simulink model "step5_forward_dyn_kine"  (Simulink 10.2)
settings: Solver=FixedStepAuto  StartTime=0.0  StopTime=3  FixedStep=T_step  RelTol=1e-3
values from neighbouring files (symbols this model uses):
  Coefddq1 = polyfit(tv,ddq1d,5)    [TrajectoryPlanning_simulink.m]    (also in step2.mat = [4.72491967588e-15 -3.27046494167e-13 33.9277839628 -50.8916; step2_trajectory.m = polyfit(t_action,ddq1d,5); step3.m)
  Coefddq2 = polyfit(tv,ddq2d,5)    [TrajectoryPlanning_simulink.m]    (also in step2.mat = [9.35976668804e-13 -4.53899397056e-12 272.296235919 -408.444; step2_trajectory.m = polyfit(t_action,ddq2d,5); step3.m)
  Coefddq3 = polyfit(tv,ddq3d,5)    [TrajectoryPlanning_simulink.m]    (also in step2.mat = [-8.62483792285e-13 3.31083832504e-12 -180.560313738 270.840; step2_trajectory.m = polyfit(t_action,ddq3d,5); step3.m)
  Coefdq1 = polyfit(tv,dq1d,5)    [TrajectoryPlanning_simulink.m]    (also in step2.mat = [-5.68315943596e-14 8.48194599071 -16.9638919814 8.481945990; step2_trajectory.m = polyfit(t_action,dq1d,5); step3.m)
  Coefdq2 = polyfit(tv,dq2d,5)    [TrajectoryPlanning_simulink.m]    (also in step2.mat = [-5.14425222069e-13 68.0740589798 -136.14811796 68.074058979; step2_trajectory.m = polyfit(t_action,dq2d,5); step3.m)
  Coefdq3 = polyfit(tv,dq3d,5)    [TrajectoryPlanning_simulink.m]    (also in step2.mat = [8.05653713588e-13 -45.1400784346 90.2801568692 -45.14007843; step2_trajectory.m = polyfit(t_action,dq3d,5); step3.m)
  Coefq1 = polyfit(tv,q1d,5)    [TrajectoryPlanning_simulink.m]    (also in step2.mat = [1.69638919814 -4.24097299536 2.82731533024 7.50224544818e-1; step2_trajectory.m = polyfit(t_action,q1d,5); step3.m)
  Coefq2 = polyfit(tv,q2d,5)    [TrajectoryPlanning_simulink.m]    (also in step2.mat = [13.614811796 -34.0370294899 22.6913529933 -2.13681015439e-1; step2_trajectory.m = polyfit(t_action,q2d,5); step3.m)
  Coefq3 = polyfit(tv,q3d,5)    [TrajectoryPlanning_simulink.m]    (also in step2.mat = [-9.02801568692 22.5700392173 -15.0466928115 8.32884443522e-; step2_trajectory.m = polyfit(t_action,q3d,5); step3.m)
  F = [Fx;Fy;Mz]    [Jacobi_T.m]    (also in PRBDM_CTC_task.m = M_tilda*v+C_tilda*dX+G_tilda; RRR_CTC_task.m = M_tilda*v+V_tilda*dX+G_tilda; RRR_jtraj.m = q0; step2.mat = 10)
  gama0 = Rparams4dyn(3)    [PRBDM_3R_Dynamic_Matrices_Lagrange.m]    (also in PRBDM_3R_Dynamics.m = in4dyn(12); PRBDM_3R_Dynamics00.m = in4dyn(12); PRBDM_3R_DynamicsPID.m = in4dyn(12); PRBDM_3R_parameters.m = 0.1)
  gama1 = x(7)    [Jacobi_T.m]    (also in PRBDM_3R_Dynamic_Matrices_Lagrange.m = Rparams4dyn(4); PRBDM_3R_Dynamics.m = in4dyn(13); PRBDM_3R_Dynamics00.m = in4dyn(13); PRBDM_3R_DynamicsPID.m = in4dyn(13))
  gama2 = x(8)    [Jacobi_T.m]    (also in PRBDM_3R_Dynamic_Matrices_Lagrange.m = Rparams4dyn(5); PRBDM_3R_Dynamics.m = in4dyn(14); PRBDM_3R_Dynamics00.m = in4dyn(14); PRBDM_3R_DynamicsPID.m = in4dyn(14))
  gama3 = x(9)    [Jacobi_T.m]    (also in PRBDM_3R_Dynamic_Matrices_Lagrange.m = Rparams4dyn(6); PRBDM_3R_Dynamics.m = in4dyn(15); PRBDM_3R_Dynamics00.m = in4dyn(15); PRBDM_3R_DynamicsPID.m = in4dyn(15))
  I = Rparams4dyn(10)    [PRBDM_3R_Dynamic_Matrices_Lagrange.m]    (also in PRBDM_3R_Dynamics.m = in4dyn(19); PRBDM_3R_Dynamics00.m = in4dyn(19); PRBDM_3R_DynamicsPID.m = in4dyn(19); PRBDM_3R_parameters.m = 1.8e-11)
  k1 = Rparams4dyn(7)    [PRBDM_3R_Dynamic_Matrices_Lagrange.m]    (also in PRBDM_3R_Dynamics.m = in4dyn(16); PRBDM_3R_Dynamics00.m = in4dyn(16); PRBDM_3R_DynamicsPID.m = in4dyn(16); PRBDM_3R_parameters.m = 0.290628)
  k2 = Rparams4dyn(8)    [PRBDM_3R_Dynamic_Matrices_Lagrange.m]    (also in PRBDM_3R_Dynamics.m = in4dyn(17); PRBDM_3R_Dynamics00.m = in4dyn(17); PRBDM_3R_DynamicsPID.m = in4dyn(17); PRBDM_3R_parameters.m = 0.247572)
  k3 = Rparams4dyn(9)    [PRBDM_3R_Dynamic_Matrices_Lagrange.m]    (also in PRBDM_3R_Dynamics.m = in4dyn(18); PRBDM_3R_Dynamics00.m = in4dyn(18); PRBDM_3R_DynamicsPID.m = in4dyn(18); PRBDM_3R_parameters.m = 0.213624)
  L = Rparams4dyn(2)    [PRBDM_3R_Dynamic_Matrices_Lagrange.m]    (also in PRBDM_3R_Dynamics.m = in4dyn(11); PRBDM_3R_Dynamics00.m = in4dyn(11); PRBDM_3R_DynamicsPID.m = in4dyn(11); PRBDM_3R_parameters.m = 0.3)
  L0 = z(7)    [Forward_kinematics.m]    (also in GeometricCalculation_simulink.m = Geoparams(4); PRBDM_3R_parameters.m = 0.03; PRBDM_3R_parameters.mat = 0.03; TrajectoryPlanning_simulink.m = X(8))
  L1 = z(8)    [Forward_kinematics.m]    (also in GeometricCalculation_simulink.m = Geoparams(5); Jacobi.m = x(4); PRBDM_3R_CTC.m = x(19); PRBDM_3R_Dynamic_Matrices_NewtonEular.m = robot_params(4))
  L2 = z(9)    [Forward_kinematics.m]    (also in GeometricCalculation_simulink.m = Geoparams(6); Jacobi.m = x(5); PRBDM_3R_CTC.m = x(20); PRBDM_3R_Dynamic_Matrices_NewtonEular.m = robot_params(5))
  L3 = z(10)    [Forward_kinematics.m]    (also in GeometricCalculation_simulink.m = Geoparams(7); Jacobi.m = x(6); PRBDM_3R_CTC.m = x(21); PRBDM_3R_Dynamic_Matrices_NewtonEular.m = robot_params(6))
  m = Rparams4dyn(1)    [PRBDM_3R_Dynamic_Matrices_Lagrange.m]    (also in PRBDM_3R_Dynamics.m = in4dyn(10); PRBDM_3R_Dynamics00.m = in4dyn(10); PRBDM_3R_DynamicsPID.m = in4dyn(10); PRBDM_3R_parameters.m = 1)
  Mz = x(6)    [Jacobi_T.m]    (also in step2.mat = 10; step2_trajectory.m = 10; step3.m = 10)
  phi_f = 1.0471975512    [step2.mat]    (also in step2_trajectory.m; step3.m)
  T_action = 1    [step2.mat]    (also in step2_trajectory.m)
  Theta_init = [0 0 0 0]    [step2.mat]    (also in step2_trajectory.m = [0     0     0     0    ]; step3.m = [0     0     0     0    ])
  W = x(22)    [PRBDM_3R_CTC.m]    (also in PRBDM_3R_Dynamic_Matrices_NewtonEular.m = robot_params(7); PRBDM_3R_Dynamics.m = in4dyn(20); PRBDM_3R_Dynamics00.m = in4dyn(20); PRBDM_3R_DynamicsPID.m = in4dyn(20))
  x_f = 0.0536    [step2.mat]    (also in step2_trajectory.m; step3.m)
  y_f = 0.135    [step2.mat]    (also in step2_trajectory.m; step3.m)
settings Model: Creator=Master  LastModifiedBy=Master
settings SolverCC: AlgebraicLoopSolver=LineSearch
settings DataIOCC: SaveFormat=Dataset  SignalLoggingSaveFormat=Dataset  ReturnWorkspaceOutputs=on
settings OptimizationCC: LifeSpan=auto
settings DebuggingCC: UnderspecifiedInitializationDetection=Simplified  MergeDetectMultiDrivingBlocksExec=error  FcnCallInpInsideContextMsg=error  SFUnexpectedBacktrackingDiag=error  SFNoUnconditionalDefaultTransitionDiag=error  SFExecutionAtInitializationDiag=warning  UnderSpecifiedDimensionMsg=error  ArithmeticOperatorsInVariantConditions=error
settings HardwareCC: ProdBitPerPointer=64  ProdBitPerSizeT=64  ProdBitPerPtrDiffT=64  ProdLargestAtomicFloat=Float  ProdIntDivRoundTo=Zero  ProdEndianess=LittleEndian  ProdWordSize=64  ProdHWDeviceType=Intel->x86-64 (Windows64)
settings ModelReferenceCC: PropagateSignalLabelsOutOfModel=on
settings SFSimCC: SimUseLocalCustomCode=on  CustomCodeUndefinedFunction=FilterOut
settings RTWCC: RTWUseLocalCustomCode=on
settings CodeAppCC: StateflowObjectComments=off
settings GRTTargetCC: TargetLangStandard=C99 (ISO)  CombineOutputUpdateFcns=on  GRTInterface=off
settings ConfigComp: CovMetricSettings=dwe  CovSaveCumulativeToWorkspaceVar=off  CovSaveSingleToWorkspaceVar=off  CovExternalEMLEnable=on

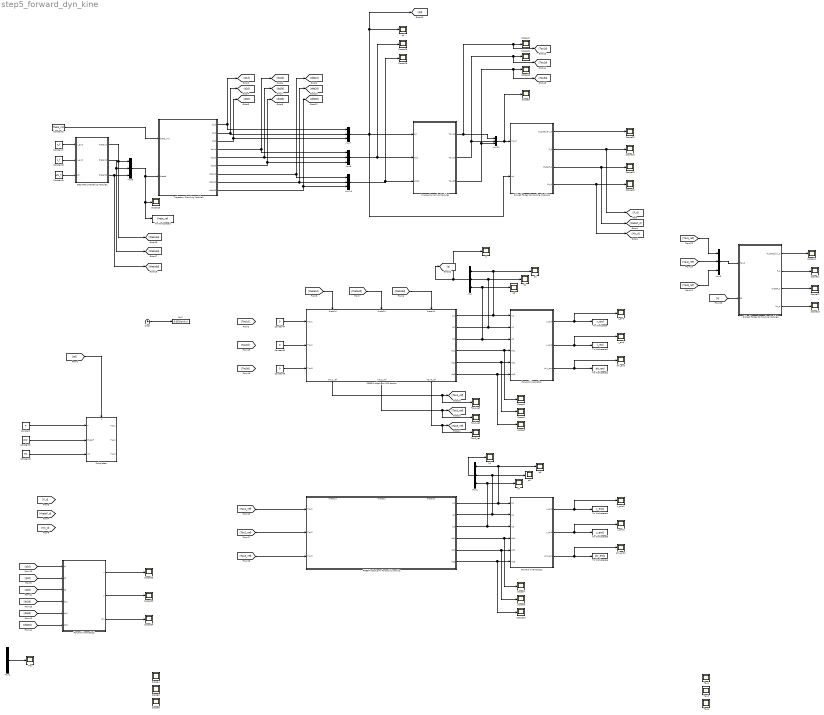
== system step5_forward_dyn_kine ==
  Clock : Clock
  Constant : Constant  Value=F
  Constant1 : Constant  Value=pi/2
  Constant2 : Constant  Value=Theta_init
  Constant3 : Constant  Value=Mz
  Constant4 : Constant  Value=0
  Constant5 : Constant  Value=0
  Constant6 : Constant  Value=0
  Constant7 : Constant  Value=x_f
  Constant8 : Constant  Value=y_f
  Constant9 : Constant  Value=phi_f
  Disired Forces Computing Module1 : Subsystem
  Disired Forces Computing Module2 : Subsystem
  Fcn7 : Fcn  Expr=0.001*sin(u)
  Forward kinematics : Subsystem
  Forward kinematics1 : Subsystem
  Forward kinematics2 : Subsystem
  Geometric Modeling Module1 : Subsystem
  Inverse Dynamics Module1 : Subsystem
  Mux{,1,3,7..11} (8 alike) : Mux  Inputs=3
  Mux2 : Mux  Inputs=6
  PRBDM robot arm Forward dynamics : Subsystem
      settings: PortSchema="{\"entries\":[{\"content\":{\"sides\":[{\"content\":{\"connectorIds\":[\"In1\",\"In2\",\"In3\"]},\"type\":\"ConnectorPlacement.EquallySpacedRectSide\",\"uuid\":\"1f88892b-0bd0-49de-aca9-2c32e7693572\"},{\"content\":{\"connectorIds\":[\"Out1\",\"Out2\",\"Out3\",\"Out4\",\"Out5\",\"Out6\"],\"side\":\"RIGHT\"},\"type\":\"ConnectorPlacement.EquallySpacedRectSide\",\"uuid\":\"b703a21d-fa56-4217-8064-1c2098ab3c38\"},{\"content\":{\"connectorIds\":[\"In4\",\"In5\",\"In6\"],\"side\":\"TOP\"},\"type\":\"ConnectorPlacement.EquallySpacedRectSide\",\"uuid\":\"2526ef97-18a1-4ac3-963d-0ba7d1a2d319\"},{\"content\":{\"connectorIds\":[],\"side\":\"BOTTOM\"},\"type\":\"ConnectorPlacement.EquallySpacedRectSide\",\"uuid\":\"f33fbcfd-8e0b-408f-a669-776188a4cff3\"},{\"content\":{\"connectorIds\":[],\"side\":\"HIDDEN\"},\"type\":\"ConnectorPlacement.EquallySpacedRectSide\",\"uuid\":\"8c9044ff-40c0-4995-b32e-bf50be4b71db\"}]},\"type\":\"ConnectorPlacement.EquallySpacedConnector\",\"uuid\":\"32b5ad01-d59a-45fa-aad8-e0a4c9d304fb\"}],\"packageUris\":[\"http://schema.mathworks.com/mf0/Connector/R2020b\"],\"version\":\"1.0\"}"
      mask Display: image(imread('RRR.png'))
  PRBDM robot arm PID control : Subsystem
      settings: PortSchema="{\"entries\":[{\"content\":{\"sides\":[{\"content\":{\"connectorIds\":[\"In1\",\"In2\",\"In3\"]},\"type\":\"ConnectorPlacement.EquallySpacedRectSide\",\"uuid\":\"1f88892b-0bd0-49de-aca9-2c32e7693572\"},{\"content\":{\"connectorIds\":[\"Out1\",\"Out2\",\"Out3\",\"Out4\",\"Out5\",\"Out6\"],\"side\":\"RIGHT\"},\"type\":\"ConnectorPlacement.EquallySpacedRectSide\",\"uuid\":\"b703a21d-fa56-4217-8064-1c2098ab3c38\"},{\"content\":{\"connectorIds\":[\"In4\",\"In5\",\"In6\"],\"side\":\"TOP\"},\"type\":\"ConnectorPlacement.EquallySpacedRectSide\",\"uuid\":\"2526ef97-18a1-4ac3-963d-0ba7d1a2d319\"},{\"content\":{\"connectorIds\":[\"Out7\",\"Out8\",\"Out9\"],\"side\":\"BOTTOM\"},\"type\":\"ConnectorPlacement.EquallySpacedRectSide\",\"uuid\":\"f33fbcfd-8e0b-408f-a669-776188a4cff3\"},{\"content\":{\"connectorIds\":[],\"side\":\"HIDDEN\"},\"type\":\"ConnectorPlacement.EquallySpacedRectSide\",\"uuid\":\"8c9044ff-40c0-4995-b32e-bf50be4b71db\"}]},\"type\":\"ConnectorPlacement.EquallySpacedConnector\",\"uuid\":\"32b5ad01-d59a-45fa-aad8-e0a4c9d304fb\"}],\"packageUris\":[\"http://schema.mathworks.com/mf0/Connector/R2020b\"],\"version\":\"1.0\"}"
      mask Display: image(imread('RRR.png'))
  Scope{1..14,16..23,25..26,33..35} (27 alike) : Scope
  Subsystem : Subsystem
      settings: PortSchema="{\"entries\":[{\"content\":{\"sides\":[{\"content\":{\"connectorIds\":[\"In1\",\"In2\",\"In3\"]},\"type\":\"ConnectorPlacement.EquallySpacedRectSide\",\"uuid\":\"03e3fa68-98df-40a7-88fb-f274e89646de\"},{\"content\":{\"connectorIds\":[\"Out1\",\"Out2\",\"Out3\"],\"side\":\"RIGHT\"},\"type\":\"ConnectorPlacement.EquallySpacedRectSide\",\"uuid\":\"1a7c6e69-d785-4f03-b0d8-74a38f8f42a1\"},{\"content\":{\"connectorIds\":[\"In4\"],\"side\":\"TOP\"},\"type\":\"ConnectorPlacement.EquallySpacedRectSide\",\"uuid\":\"61c135cb-8cc5-493d-9c37-8230cda997e1\"},{\"content\":{\"connectorIds\":[],\"side\":\"HIDDEN\"},\"type\":\"ConnectorPlacement.EquallySpacedRectSide\",\"uuid\":\"5d99950e-feb6-474c-993a-cad470b06503\"}]},\"type\":\"ConnectorPlacement.EquallySpacedConnector\",\"uuid\":\"5533c5e9-db4a-4e3a-8115-8d67f8979e0c\"}],\"packageUris\":[\"http://schema.mathworks.com/mf0/Connector/R2020b\"],\"version\":\"1.0\"}"
  Tau{,4..6} (4 alike) : Scope
  Tau1_ref : Scope
  Tau2_ref : Scope
  Tau3_ref : Scope
  To Workspace : ToWorkspace  VariableName=x_end  SampleTime=-1
  To Workspace1 : ToWorkspace  VariableName=y_end  SampleTime=-1
  To Workspace2 : ToWorkspace  VariableName=phi_end  SampleTime=-1
  To Workspace3 : ToWorkspace  VariableName=theta_ref  SaveFormat=Timeseries  SampleTime=-1
  To Workspace4 : ToWorkspace  VariableName=x_end1  SampleTime=-1
  To Workspace5 : ToWorkspace  VariableName=y_end1  SampleTime=-1
  To Workspace6 : ToWorkspace  VariableName=phi_end1  SampleTime=-1
  Trajectory Planning Module1 : Subsystem
  phi_end : Scope
  phi_end1 : Scope
  q{,1..7} (8 alike) : Scope
  qd : Scope
  x_end : Scope
  x_end1 : Scope
  y_end : Scope
  y_end1 : Scope
  wires:
  Disired Forces Computing Module1/1(F_cartesian_d) -> Scope23/1
  Constant8/1 -> Geometric Modeling Module1/2(y_end)
  Trajectory Planning Module1/6(dq3d) -> [dq3d], Mux8/3
  Trajectory Planning Module1/9(ddq3d) -> [ddq3d], Mux10/3
  Trajectory Planning Module1/8(ddq2d) -> Mux10/2, [ddq2d]
  Constant9/1 -> Geometric Modeling Module1/3(phi)
  Trajectory Planning Module1/2(q2d) -> Mux7/2, [q2d]
  Trajectory Planning Module1/3(q3d) -> Mux7/3, [q3d]
  Mux11/1 -> Scope8/1, Disired Forces Computing Module1/1(Taud)
  Geometric Modeling Module1/2(theta2d) -> [theta2d], Mux9/2
  Geometric Modeling Module1/1(theta1d) -> [theta1d], Mux9/1
  Mux10/1 -> Inverse Dynamics Module1/3(ddqd), Scope26/1
  Geometric Modeling Module1/3(theta3d) -> [theta3d], Mux9/3
  Mux8/1 -> Inverse Dynamics Module1/2(dqd), Scope25/1
  Trajectory Planning Module1/1(q1d) -> Mux7/1, [q1d]
  Mux9/1 -> To Workspace3/1, Scope16/1, Trajectory Planning Module1/2(thetad)
  Constant7/1 -> Geometric Modeling Module1/1(x_end)
  Constant2/1 -> Trajectory Planning Module1/1(theta_init)
  Inverse Dynamics Module1/1(Tau1d) -> Mux11/1, [Tau1d], Scope17/1
  Inverse Dynamics Module1/2(Tau2d) -> Mux11/2, [Tau2d], Scope21/1
  PRBDM robot arm PID control/3(q3) -> q3/1, Mux/3, Forward kinematics/3(q3)
  PRBDM robot arm PID control/2(q2) -> q2/1, Mux/2, Forward kinematics/2(q2)
  PRBDM robot arm PID control/1(q1) -> Mux/1, q1/1, Forward kinematics/1(q1)
  Forward kinematics/1(x_end) -> To Workspace/1, x_end/1
  Forward kinematics/2(y_end) -> y_end/1, To Workspace1/1
  Forward kinematics/3(phi_end) -> phi_end/1, To Workspace2/1
  Disired Forces Computing Module1/2(F_d) -> [F_d], Scope18/1
  Disired Forces Computing Module1/3(thetaF_d) -> [thetaF_d], Scope19/1
  Disired Forces Computing Module1/4(Mz_d) -> [Mz_d], Scope20/1
  PRBDM robot arm PID control/4(dq1) -> Scope1/1, Forward kinematics/4(dq1)
  PRBDM robot arm PID control/5(dq2) -> Scope2/1, Forward kinematics/5(dq2)
  PRBDM robot arm PID control/6(dq3) -> Scope3/1, Forward kinematics/6(dq3)
  Trajectory Planning Module1/4(dq1d) -> Mux8/1, [dq1d]
  Trajectory Planning Module1/5(dq2d) -> [dq2d], Mux8/2
  Mux7/1 -> Disired Forces Computing Module1/2(qd), Inverse Dynamics Module1/1(qd), [qd], qd/1
  Trajectory Planning Module1/7(ddq1d) -> Mux10/1, [ddq1d]
  Clock/1 -> Fcn7/1
  Inverse Dynamics Module1/3(Tau3d) -> Mux11/3, [Tau3d], Scope22/1
  [qd] -> Subsystem/4(q)
  Mux/1 -> q/1, [q]
  [q1d] -> Forward kinematics2/1(q1)
  [q2d] -> Forward kinematics2/2(q2)
  [q3d] -> Forward kinematics2/3(q3)
  [dq1d] -> Forward kinematics2/4(dq1)
  [dq2d] -> Forward kinematics2/5(dq2)
  [ddq3d] -> Forward kinematics2/6(dq3)
  Forward kinematics2/1(x) -> Scope35/1
  Forward kinematics2/2(y) -> Scope33/1
  Forward kinematics2/3(phi) -> Scope34/1
  Mux2/1 -> Tau/1
  Constant/1 -> Subsystem/1(F)
  Constant1/1 -> Subsystem/2(thetaF)
  Constant3/1 -> Subsystem/3(Mz)
  Constant4/1 -> PRBDM robot arm PID control/1(Tau1)
  Constant5/1 -> PRBDM robot arm PID control/2(Tau2)
  Constant6/1 -> PRBDM robot arm PID control/3(Tau3)
  [theta1d] -> PRBDM robot arm PID control/4(theta1d)
  [theta2d] -> PRBDM robot arm PID control/5(theta2d)
  [theta3d] -> PRBDM robot arm PID control/6(theta3d)
  PRBDM robot arm PID control/7(Tau1_ref) -> Tau1_ref/1, [Tau1_ref]
  PRBDM robot arm PID control/8(Tau2_ref) -> Tau2_ref/1, [Tau2_ref]
  PRBDM robot arm PID control/9(Tau3_ref) -> Tau3_ref/1, [Tau3_ref]
  Mux1/1 -> q4/1
  PRBDM robot arm Forward dynamics/5(dq2) -> Scope9/1, Forward kinematics1/5(dq2)
  PRBDM robot arm Forward dynamics/1(q1) -> Mux1/1, q5/1, Forward kinematics1/1(q1)
  PRBDM robot arm Forward dynamics/6(dq3) -> Scope10/1, Forward kinematics1/6(dq3)
  PRBDM robot arm Forward dynamics/4(dq1) -> Scope7/1, Forward kinematics1/4(dq1)
  Forward kinematics1/1(x_end) -> To Workspace4/1, x_end1/1
  PRBDM robot arm Forward dynamics/2(q2) -> q6/1, Mux1/2, Forward kinematics1/2(q2)
  Forward kinematics1/3(phi_end) -> phi_end1/1, To Workspace6/1
  Forward kinematics1/2(y_end) -> y_end1/1, To Workspace5/1
  PRBDM robot arm Forward dynamics/3(q3) -> q7/1, Mux1/3, Forward kinematics1/3(q3)
  [Tau3_ref] -> PRBDM robot arm Forward dynamics/3(Tau3)
  [Tau2_ref] -> PRBDM robot arm Forward dynamics/2(Tau2)
  [Tau1_ref] -> PRBDM robot arm Forward dynamics/1(Tau1)
  [Tau2_ref] -> Mux3/2
  [Tau1_ref] -> Mux3/1
  [Tau3_ref] -> Mux3/3
  Mux3/1 -> Disired Forces Computing Module2/1(Taud)
  [q] -> Disired Forces Computing Module2/2(qd)
  Disired Forces Computing Module2/1(F_cartesian_d) -> Scope14/1
  Disired Forces Computing Module2/2(F_d) -> Scope11/1
  Disired Forces Computing Module2/4(Mz_d) -> Scope13/1
  Disired Forces Computing Module2/3(thetaF_d) -> Scope12/1

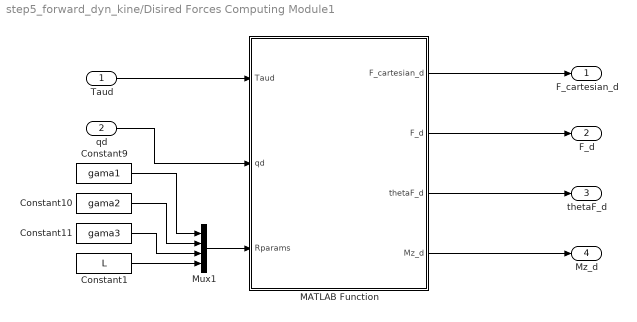
== system step5_forward_dyn_kine/Disired Forces Computing Module1 ==
  Taud : Inport
  qd : Inport  Port=2
  Constant1 : Constant  Value=L
  Constant10 : Constant  Value=gama2
  Constant11 : Constant  Value=gama3
  Constant9 : Constant  Value=gama1
  MATLAB Function : MATLAB Function  TreatAsAtomicUnit=on
  Mux1 : Mux
  F_cartesian_d : Outport
  F_d : Outport  Port=2
  thetaF_d : Outport  Port=3
  Mz_d : Outport  Port=4
  wires:
  MATLAB Function/1(F_cartesian_d) -> F_cartesian_d/1
  Mux1/1 -> MATLAB Function/3(Rparams)
  Constant9/1 -> Mux1/1
  Constant10/1 -> Mux1/2
  Constant11/1 -> Mux1/3
  Taud/1 -> MATLAB Function/1(Taud)
  qd/1 -> MATLAB Function/2(qd)
  Constant1/1 -> Mux1/4
  MATLAB Function/2(F_d) -> F_d/1
  MATLAB Function/3(thetaF_d) -> thetaF_d/1
  MATLAB Function/4(Mz_d) -> Mz_d/1

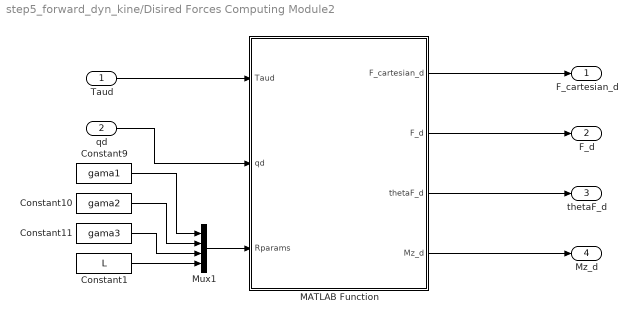
== system step5_forward_dyn_kine/Disired Forces Computing Module2 ==
  Taud : Inport
  qd : Inport  Port=2
  Constant1 : Constant  Value=L
  Constant10 : Constant  Value=gama2
  Constant11 : Constant  Value=gama3
  Constant9 : Constant  Value=gama1
  MATLAB Function : MATLAB Function  TreatAsAtomicUnit=on
  Mux1 : Mux
  F_cartesian_d : Outport
  F_d : Outport  Port=2
  thetaF_d : Outport  Port=3
  Mz_d : Outport  Port=4
  wires:
  MATLAB Function/1(F_cartesian_d) -> F_cartesian_d/1
  Mux1/1 -> MATLAB Function/3(Rparams)
  Constant9/1 -> Mux1/1
  Constant10/1 -> Mux1/2
  Constant11/1 -> Mux1/3
  Taud/1 -> MATLAB Function/1(Taud)
  qd/1 -> MATLAB Function/2(qd)
  Constant1/1 -> Mux1/4
  MATLAB Function/2(F_d) -> F_d/1
  MATLAB Function/3(thetaF_d) -> thetaF_d/1
  MATLAB Function/4(Mz_d) -> Mz_d/1

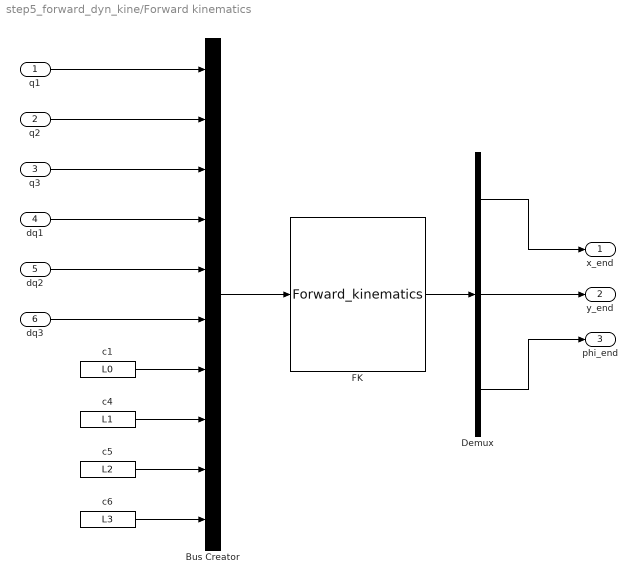
== system step5_forward_dyn_kine/Forward kinematics ==
  q1 : Inport
  q2 : Inport  Port=2
  q3 : Inport  Port=3
  dq1 : Inport  Port=4
  dq2 : Inport  Port=5
  dq3 : Inport  Port=6
  Bus Creator : BusCreator  Inputs=10
  Demux : Demux  Outputs=3
  FK : MATLABFcn  MATLABFcn=Forward_kinematics  OutputDimensions=3
  c1 : Constant  Value=L0
  c4 : Constant  Value=L1
  c5 : Constant  Value=L2
  c6 : Constant  Value=L3
  x_end : Outport
  y_end : Outport  Port=2
  phi_end : Outport  Port=3
  wires:
  c6/1 -> Bus Creator/10
  Demux/1 -> x_end/1
  c4/1 -> Bus Creator/8
  q2/1 -> Bus Creator/2
  q1/1 -> Bus Creator/1
  q3/1 -> Bus Creator/3
  Bus Creator/1 -> FK/1
  dq2/1 -> Bus Creator/5
  Demux/2 -> y_end/1
  FK/1 -> Demux/1
  dq1/1 -> Bus Creator/4
  Demux/3 -> phi_end/1
  dq3/1 -> Bus Creator/6
  c5/1 -> Bus Creator/9
  c1/1 -> Bus Creator/7

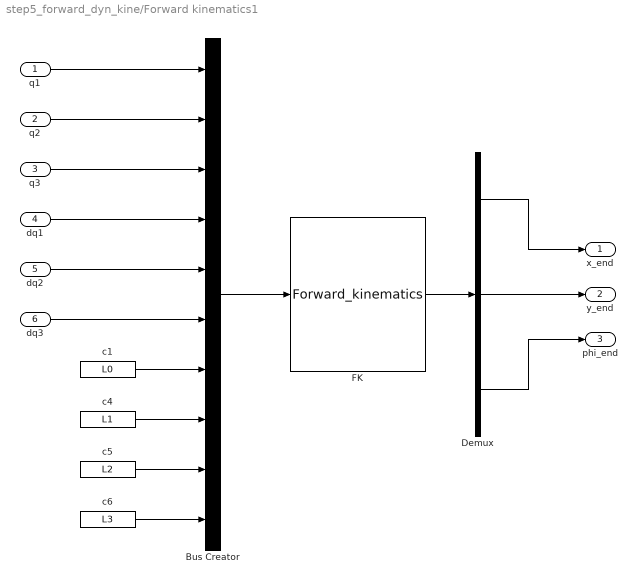
== system step5_forward_dyn_kine/Forward kinematics1 ==
  q1 : Inport
  q2 : Inport  Port=2
  q3 : Inport  Port=3
  dq1 : Inport  Port=4
  dq2 : Inport  Port=5
  dq3 : Inport  Port=6
  Bus Creator : BusCreator  Inputs=10
  Demux : Demux  Outputs=3
  FK : MATLABFcn  MATLABFcn=Forward_kinematics  OutputDimensions=3
  c1 : Constant  Value=L0
  c4 : Constant  Value=L1
  c5 : Constant  Value=L2
  c6 : Constant  Value=L3
  x_end : Outport
  y_end : Outport  Port=2
  phi_end : Outport  Port=3
  wires:
  c6/1 -> Bus Creator/10
  Demux/1 -> x_end/1
  c4/1 -> Bus Creator/8
  q2/1 -> Bus Creator/2
  q1/1 -> Bus Creator/1
  q3/1 -> Bus Creator/3
  Bus Creator/1 -> FK/1
  dq2/1 -> Bus Creator/5
  Demux/2 -> y_end/1
  FK/1 -> Demux/1
  dq1/1 -> Bus Creator/4
  Demux/3 -> phi_end/1
  dq3/1 -> Bus Creator/6
  c5/1 -> Bus Creator/9
  c1/1 -> Bus Creator/7

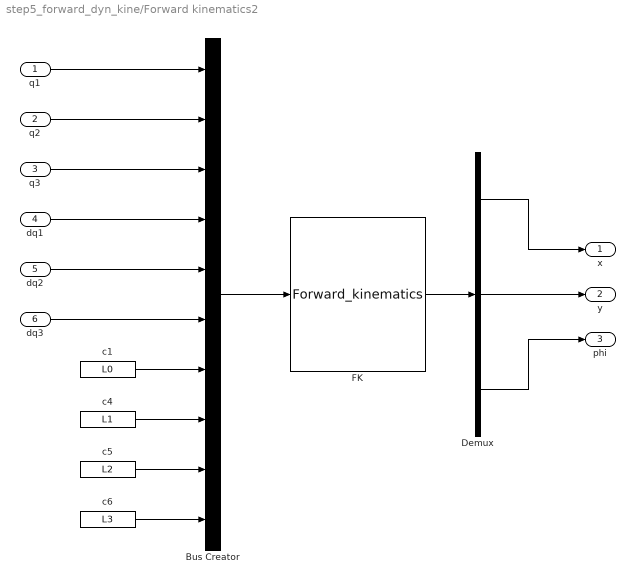
== system step5_forward_dyn_kine/Forward kinematics2 ==
  q1 : Inport
  q2 : Inport  Port=2
  q3 : Inport  Port=3
  dq1 : Inport  Port=4
  dq2 : Inport  Port=5
  dq3 : Inport  Port=6
  Bus Creator : BusCreator  Inputs=10
  Demux : Demux  Outputs=3
  FK : MATLABFcn  MATLABFcn=Forward_kinematics  OutputDimensions=3
  c1 : Constant  Value=L0
  c4 : Constant  Value=L1
  c5 : Constant  Value=L2
  c6 : Constant  Value=L3
  x : Outport
  y : Outport  Port=2
  phi : Outport  Port=3
  wires:
  c6/1 -> Bus Creator/10
  Demux/1 -> x/1
  c4/1 -> Bus Creator/8
  q2/1 -> Bus Creator/2
  q1/1 -> Bus Creator/1
  q3/1 -> Bus Creator/3
  Bus Creator/1 -> FK/1
  dq2/1 -> Bus Creator/5
  Demux/2 -> y/1
  FK/1 -> Demux/1
  dq1/1 -> Bus Creator/4
  Demux/3 -> phi/1
  dq3/1 -> Bus Creator/6
  c5/1 -> Bus Creator/9
  c1/1 -> Bus Creator/7

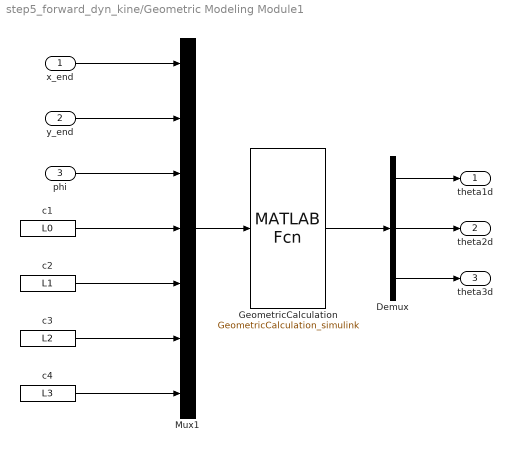
== system step5_forward_dyn_kine/Geometric Modeling Module1 ==
  x_end : Inport
  y_end : Inport  Port=2
  phi : Inport  Port=3
  Demux : Demux  Outputs=3
  GeometricCalculation : MATLABFcn  MATLABFcn=GeometricCalculation_simulink
  Mux1 : Mux  Inputs=7
  c1 : Constant  Value=L0
  c2 : Constant  Value=L1
  c3 : Constant  Value=L2
  c4 : Constant  Value=L3
  theta1d : Outport
  theta2d : Outport  Port=2
  theta3d : Outport  Port=3
  wires:
  Mux1/1 -> GeometricCalculation/1
  y_end/1 -> Mux1/2
  x_end/1 -> Mux1/1
  phi/1 -> Mux1/3
  c1/1 -> Mux1/4
  c3/1 -> Mux1/6
  c2/1 -> Mux1/5
  GeometricCalculation/1 -> Demux/1
  Demux/2 -> theta2d/1
  Demux/1 -> theta1d/1
  Demux/3 -> theta3d/1
  c4/1 -> Mux1/7

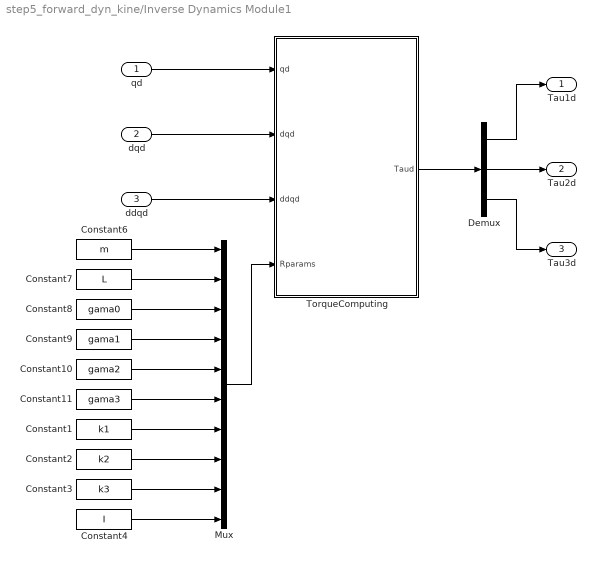
== system step5_forward_dyn_kine/Inverse Dynamics Module1 ==
  qd : Inport
  dqd : Inport  Port=2
  ddqd : Inport  Port=3
  Constant1 : Constant  Value=k1
  Constant10 : Constant  Value=gama2
  Constant11 : Constant  Value=gama3
  Constant2 : Constant  Value=k2
  Constant3 : Constant  Value=k3
  Constant4 : Constant  Value=I
  Constant6 : Constant  Value=m
  Constant7 : Constant  Value=L
  Constant8 : Constant  Value=gama0
  Constant9 : Constant  Value=gama1
  Demux : Demux  Outputs=3
  Mux : Mux  Inputs=10
  TorqueComputing : MATLAB Function  TreatAsAtomicUnit=on
  Tau1d : Outport
  Tau2d : Outport  Port=2
  Tau3d : Outport  Port=3
  wires:
  qd/1 -> TorqueComputing/1(qd)
  dqd/1 -> TorqueComputing/2(dqd)
  ddqd/1 -> TorqueComputing/3(ddqd)
  TorqueComputing/1(Taud) -> Demux/1
  Demux/2 -> Tau2d/1
  Demux/1 -> Tau1d/1
  Demux/3 -> Tau3d/1
  Mux/1 -> TorqueComputing/4(Rparams)
  Constant6/1 -> Mux/1
  Constant7/1 -> Mux/2
  Constant8/1 -> Mux/3
  Constant9/1 -> Mux/4
  Constant10/1 -> Mux/5
  Constant11/1 -> Mux/6
  Constant1/1 -> Mux/7
  Constant2/1 -> Mux/8
  Constant3/1 -> Mux/9
  Constant4/1 -> Mux/10

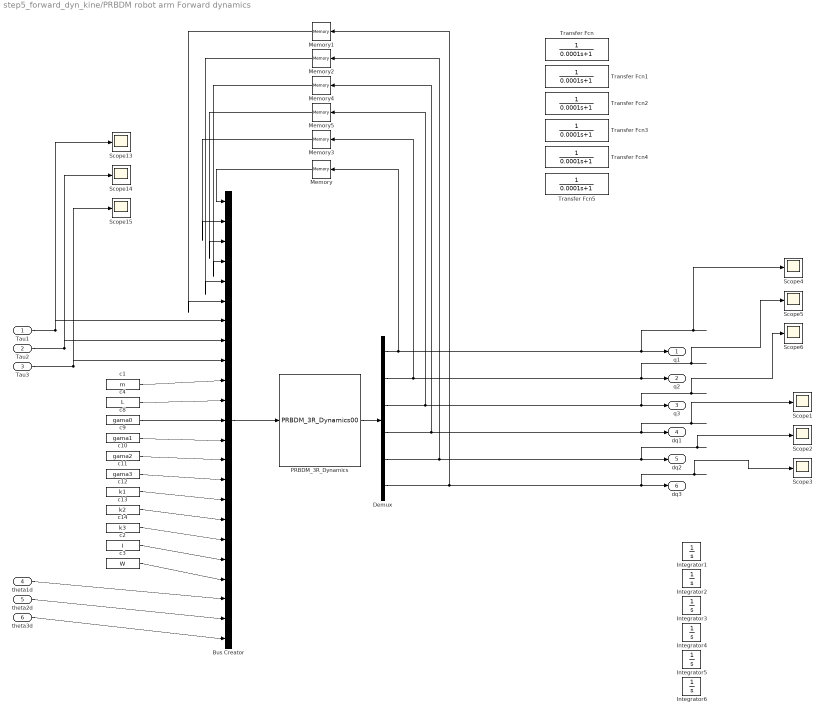
== system step5_forward_dyn_kine/PRBDM robot arm Forward dynamics ==
  Tau1 : Inport
  Tau2 : Inport  Port=2
  Tau3 : Inport  Port=3
  theta1d : Inport  Port=4
  theta2d : Inport  Port=5
  theta3d : Inport  Port=6
  Bus Creator : BusCreator  Inputs=23
  Demux : Demux  Outputs=6
  Integrator{1..6} (6 alike) : Integrator  UpperSaturationLimit=1e6  LowerSaturationLimit=-1e6
  Memory{,1..5} (6 alike) : Memory
  PRBDM_3R_Dynamics : MATLABFcn  MATLABFcn=PRBDM_3R_Dynamics00  OutputDimensions=6
  Scope{1..6,13..15} (9 alike) : Scope
  Transfer Fcn{,1..5} (6 alike) : TransferFcn  Denominator=[0.0001 1]
  c1 : Constant  Value=m
  c10 : Constant  Value=gama2
  c11 : Constant  Value=gama3
  c12 : Constant  Value=k1
  c13 : Constant  Value=k2
  c14 : Constant  Value=k3
  c2 : Constant  Value=I
  c3 : Constant  Value=W
  c4 : Constant  Value=L
  c8 : Constant  Value=gama0
  c9 : Constant  Value=gama1
  q1 : Outport
  q2 : Outport  Port=2
  q3 : Outport  Port=3
  dq1 : Outport  Port=4
  dq2 : Outport  Port=5
  dq3 : Outport  Port=6
  wires:
  theta3d/1 -> Bus Creator/23
  theta2d/1 -> Bus Creator/22
  c11/1 -> Bus Creator/15
  c3/1 -> Bus Creator/20
  c14/1 -> Bus Creator/18
  c2/1 -> Bus Creator/19
  c1/1 -> Bus Creator/10
  c8/1 -> Bus Creator/12
  Bus Creator/1 -> PRBDM_3R_Dynamics/1
  Tau1/1 -> Scope13/1, Bus Creator/7
  PRBDM_3R_Dynamics/1 -> Demux/1
  c4/1 -> Bus Creator/11
  c10/1 -> Bus Creator/14
  c9/1 -> Bus Creator/13
  c13/1 -> Bus Creator/17
  Tau3/1 -> Scope15/1, Bus Creator/9
  c12/1 -> Bus Creator/16
  theta1d/1 -> Bus Creator/21
  Tau2/1 -> Scope14/1, Bus Creator/8
  Demux/1 -> Memory/1, q1/1, Scope4/1
  Demux/2 -> Memory3/1, q2/1, Scope5/1
  Demux/3 -> Memory5/1, q3/1, Scope6/1
  Demux/4 -> Memory4/1, dq1/1, Scope1/1
  Demux/5 -> Memory2/1, dq2/1, Scope2/1
  Demux/6 -> Memory1/1, dq3/1, Scope3/1
  Memory/1 -> Bus Creator/1
  Memory3/1 -> Bus Creator/2
  Memory5/1 -> Bus Creator/3
  Memory4/1 -> Bus Creator/4
  Memory2/1 -> Bus Creator/5
  Memory1/1 -> Bus Creator/6

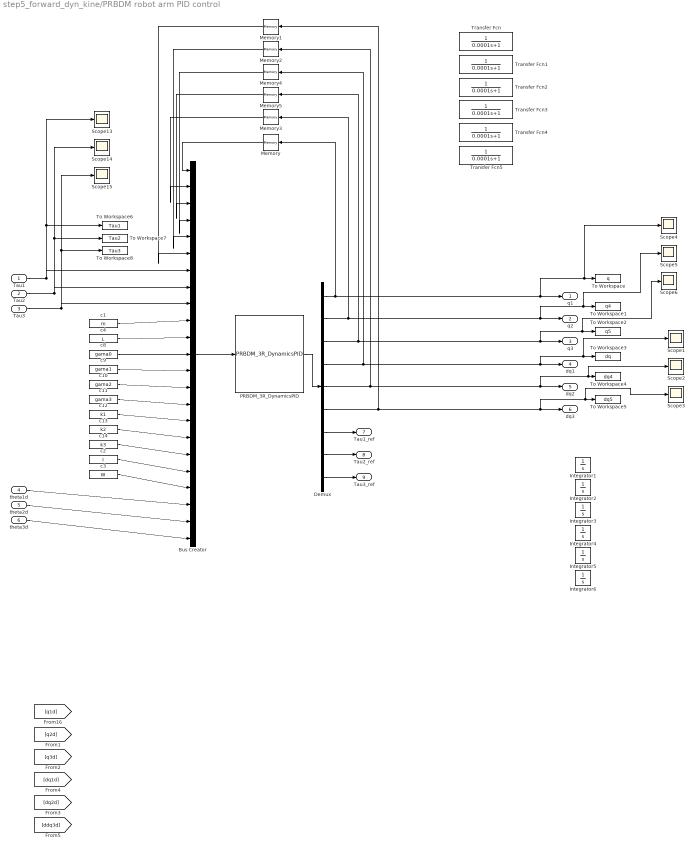
== system step5_forward_dyn_kine/PRBDM robot arm PID control ==
  Tau1 : Inport
  Tau2 : Inport  Port=2
  Tau3 : Inport  Port=3
  theta1d : Inport  Port=4
  theta2d : Inport  Port=5
  theta3d : Inport  Port=6
  Bus Creator : BusCreator  Inputs=23
  Demux : Demux  Outputs=9
  Integrator{1..6} (6 alike) : Integrator  UpperSaturationLimit=1e6  LowerSaturationLimit=-1e6
  Memory{,1..5} (6 alike) : Memory
  PRBDM_3R_DynamicsPID : MATLABFcn  MATLABFcn=PRBDM_3R_DynamicsPID  OutputDimensions=9
  Scope{1..6,13..15} (9 alike) : Scope
  To Workspace : ToWorkspace  VariableName=q  SampleTime=-1
  To Workspace1 : ToWorkspace  VariableName=q4  SampleTime=-1
  To Workspace2 : ToWorkspace  VariableName=q5  SampleTime=-1
  To Workspace3 : ToWorkspace  VariableName=dq  SampleTime=-1
  To Workspace4 : ToWorkspace  VariableName=dq4  SampleTime=-1
  To Workspace5 : ToWorkspace  VariableName=dq5  SampleTime=-1
  To Workspace6 : ToWorkspace  VariableName=Tau1  SampleTime=-1
  To Workspace7 : ToWorkspace  VariableName=Tau2  SampleTime=-1
  To Workspace8 : ToWorkspace  VariableName=Tau3  SampleTime=-1
  Transfer Fcn{,1..5} (6 alike) : TransferFcn  Denominator=[0.0001 1]
  c1 : Constant  Value=m
  c10 : Constant  Value=gama2
  c11 : Constant  Value=gama3
  c12 : Constant  Value=k1
  c13 : Constant  Value=k2
  c14 : Constant  Value=k3
  c2 : Constant  Value=I
  c3 : Constant  Value=W
  c4 : Constant  Value=L
  c8 : Constant  Value=gama0
  c9 : Constant  Value=gama1
  q1 : Outport
  q2 : Outport  Port=2
  q3 : Outport  Port=3
  dq1 : Outport  Port=4
  dq2 : Outport  Port=5
  dq3 : Outport  Port=6
  Tau1_ref : Outport  Port=7
  Tau2_ref : Outport  Port=8
  Tau3_ref : Outport  Port=9
  wires:
  theta3d/1 -> Bus Creator/23
  theta2d/1 -> Bus Creator/22
  c11/1 -> Bus Creator/15
  c3/1 -> Bus Creator/20
  c14/1 -> Bus Creator/18
  c2/1 -> Bus Creator/19
  c1/1 -> Bus Creator/10
  c8/1 -> Bus Creator/12
  Bus Creator/1 -> PRBDM_3R_DynamicsPID/1
  Tau1/1 -> To Workspace6/1, Scope13/1, Bus Creator/7
  PRBDM_3R_DynamicsPID/1 -> Demux/1
  c4/1 -> Bus Creator/11
  c10/1 -> Bus Creator/14
  c9/1 -> Bus Creator/13
  c13/1 -> Bus Creator/17
  Tau3/1 -> Scope15/1, To Workspace8/1, Bus Creator/9
  c12/1 -> Bus Creator/16
  theta1d/1 -> Bus Creator/21
  Tau2/1 -> To Workspace7/1, Scope14/1, Bus Creator/8
  Demux/1 -> Memory/1, q1/1, Scope4/1, To Workspace/1
  Demux/2 -> Memory3/1, q2/1, Scope5/1, To Workspace1/1
  Demux/3 -> Memory5/1, q3/1, Scope6/1, To Workspace2/1
  Demux/4 -> Memory4/1, dq1/1, Scope1/1, To Workspace3/1
  Demux/5 -> Memory2/1, dq2/1, Scope2/1, To Workspace4/1
  Demux/6 -> Memory1/1, dq3/1, Scope3/1, To Workspace5/1
  Memory/1 -> Bus Creator/1
  Memory3/1 -> Bus Creator/2
  Memory5/1 -> Bus Creator/3
  Memory4/1 -> Bus Creator/4
  Memory2/1 -> Bus Creator/5
  Memory1/1 -> Bus Creator/6
  Demux/7 -> Tau1_ref/1
  Demux/8 -> Tau2_ref/1
  Demux/9 -> Tau3_ref/1

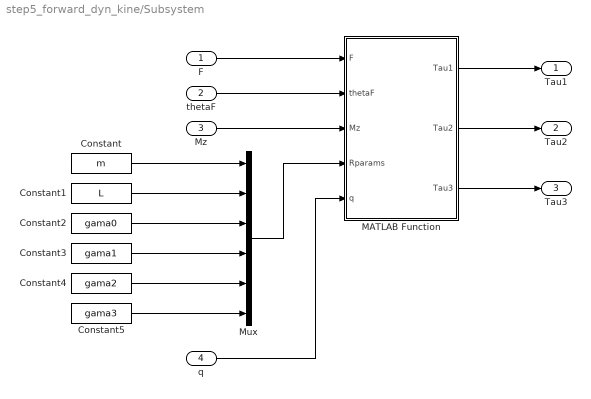
== system step5_forward_dyn_kine/Subsystem ==
  F : Inport
  thetaF : Inport  Port=2
  Mz : Inport  Port=3
  q : Inport  Port=4
  Constant : Constant  Value=m
  Constant1 : Constant  Value=L
  Constant2 : Constant  Value=gama0
  Constant3 : Constant  Value=gama1
  Constant4 : Constant  Value=gama2
  Constant5 : Constant  Value=gama3
  MATLAB Function : MATLAB Function  TreatAsAtomicUnit=on
  Mux : Mux  Inputs=6
  Tau1 : Outport
  Tau2 : Outport  Port=2
  Tau3 : Outport  Port=3
  wires:
  thetaF/1 -> MATLAB Function/2(thetaF)
  F/1 -> MATLAB Function/1(F)
  Mz/1 -> MATLAB Function/3(Mz)
  MATLAB Function/1(Tau1) -> Tau1/1
  Constant/1 -> Mux/1
  Constant1/1 -> Mux/2
  Constant2/1 -> Mux/3
  Constant3/1 -> Mux/4
  Constant4/1 -> Mux/5
  Constant5/1 -> Mux/6
  Mux/1 -> MATLAB Function/4(Rparams)
  MATLAB Function/2(Tau2) -> Tau2/1
  MATLAB Function/3(Tau3) -> Tau3/1
  q/1 -> MATLAB Function/5(q)

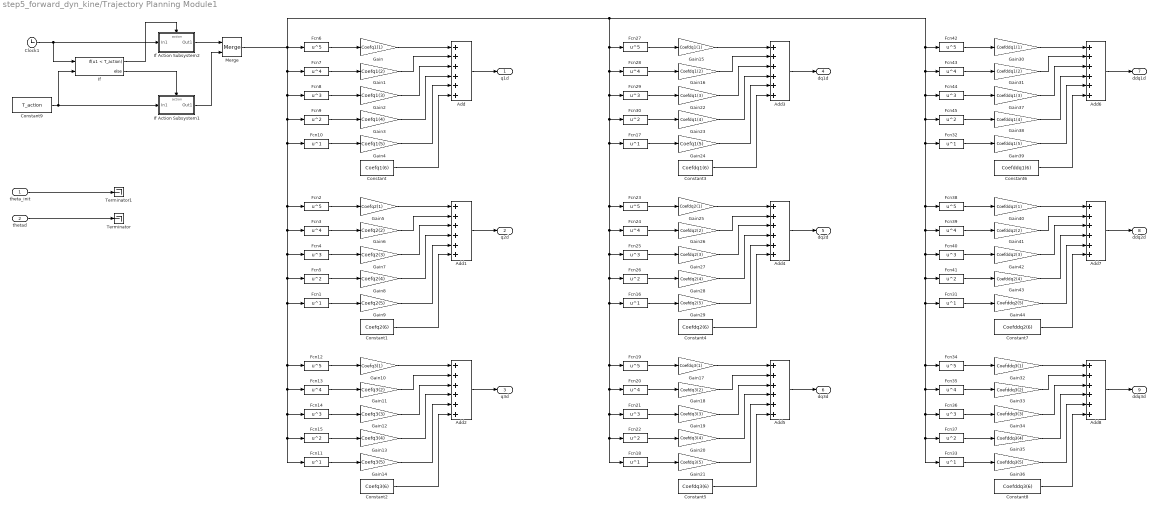
== system step5_forward_dyn_kine/Trajectory Planning Module1 ==
  theta_init : Inport
  thetad : Inport  Port=2
  Add{,1..8} (9 alike) : Sum  Inputs=++++++
  Clock1 : Clock
  Constant : Constant  Value=Coefq1(6)
  Constant1 : Constant  Value=Coefq2(6)
  Constant2 : Constant  Value=Coefq3(6)
  Constant3 : Constant  Value=Coefdq1(6)
  Constant4 : Constant  Value=Coefdq2(6)
  Constant5 : Constant  Value=Coefdq3(6)
  Constant6 : Constant  Value=Coefddq1(6)
  Constant7 : Constant  Value=Coefddq2(6)
  Constant8 : Constant  Value=Coefddq3(6)
  Constant9 : Constant  Value=T_action
  Fcn{1,10..11,16..18,31..33} (9 alike) : Fcn  Expr=u^1
  Fcn{2,6,12,19,23,27,34,38,42} (9 alike) : Fcn  Expr=u^5
  Fcn{3,7,13,20,24,28,35,39,43} (9 alike) : Fcn  Expr=u^4
  Fcn{4,8,14,21,25,29,36,40,44} (9 alike) : Fcn  Expr=u^3
  Fcn{5,9,15,22,26,30,37,41,45} (9 alike) : Fcn  Expr=u^2
  Gain : Gain  Gain=Coefq1(1)
  Gain1 : Gain  Gain=Coefq1(2)
  Gain10 : Gain  Gain=Coefq3(1)
  Gain11 : Gain  Gain=Coefq3(2)
  Gain12 : Gain  Gain=Coefq3(3)
  Gain13 : Gain  Gain=Coefq3(4)
  Gain14 : Gain  Gain=Coefq3(5)
  Gain15 : Gain  Gain=Coefdq1(1)
  Gain16 : Gain  Gain=Coefdq1(2)
  Gain17 : Gain  Gain=Coefdq3(1)
  Gain18 : Gain  Gain=Coefdq3(2)
  Gain19 : Gain  Gain=Coefdq3(3)
  Gain2 : Gain  Gain=Coefq1(3)
  Gain20 : Gain  Gain=Coefdq3(4)
  Gain21 : Gain  Gain=Coefdq3(5)
  Gain22 : Gain  Gain=Coefdq1(3)
  Gain23 : Gain  Gain=Coefdq1(4)
  Gain24 : Gain  Gain=Coefq1(5)
  Gain25 : Gain  Gain=Coefdq2(1)
  Gain26 : Gain  Gain=Coefdq2(2)
  Gain27 : Gain  Gain=Coefdq2(3)
  Gain28 : Gain  Gain=Coefdq2(4)
  Gain29 : Gain  Gain=Coefdq2(5)
  Gain3 : Gain  Gain=Coefq1(4)
  Gain30 : Gain  Gain=Coefddq1(1)
  Gain31 : Gain  Gain=Coefddq1(2)
  Gain32 : Gain  Gain=Coefddq3(1)
  Gain33 : Gain  Gain=Coefddq3(2)
  Gain34 : Gain  Gain=Coefddq3(3)
  Gain35 : Gain  Gain=Coefddq3(4)
  Gain36 : Gain  Gain=Coefddq3(5)
  Gain37 : Gain  Gain=Coefddq1(3)
  Gain38 : Gain  Gain=Coefddq1(4)
  Gain39 : Gain  Gain=Coefddq1(5)
  Gain4 : Gain  Gain=Coefq1(5)
  Gain40 : Gain  Gain=Coefddq2(1)
  Gain41 : Gain  Gain=Coefddq2(2)
  Gain42 : Gain  Gain=Coefddq2(3)
  Gain43 : Gain  Gain=Coefddq2(4)
  Gain44 : Gain  Gain=Coefddq2(5)
  Gain5 : Gain  Gain=Coefq2(1)
  Gain6 : Gain  Gain=Coefq2(2)
  Gain7 : Gain  Gain=Coefq2(3)
  Gain8 : Gain  Gain=Coefq2(4)
  Gain9 : Gain  Gain=Coefq2(5)
  If : If  NumInputs=2  IfExpression=u1 < T_action
  If Action Subsystem1 : Subsystem  TreatAsAtomicUnit=on
  If Action Subsystem2 : Subsystem  TreatAsAtomicUnit=on
  Merge : Merge
  Terminator : Terminator
  Terminator1 : Terminator
  q1d : Outport
  q2d : Outport  Port=2
  q3d : Outport  Port=3
  dq1d : Outport  Port=4
  dq2d : Outport  Port=5
  dq3d : Outport  Port=6
  ddq1d : Outport  Port=7
  ddq2d : Outport  Port=8
  ddq3d : Outport  Port=9
  wires:
  Clock1/1 -> If Action Subsystem2/1(In1), If/1
  Fcn6/1 -> Gain/1
  Fcn8/1 -> Gain2/1
  Fcn7/1 -> Gain1/1
  Fcn9/1 -> Gain3/1
  Fcn10/1 -> Gain4/1
  Gain/1 -> Add/1
  Gain1/1 -> Add/2
  Gain2/1 -> Add/3
  Gain3/1 -> Add/4
  Gain4/1 -> Add/5
  Constant/1 -> Add/6
  Add/1 -> q1d/1
  Add1/1 -> q2d/1
  Fcn2/1 -> Gain5/1
  Fcn5/1 -> Gain8/1
  Gain6/1 -> Add1/2
  Gain9/1 -> Add1/5
  Constant1/1 -> Add1/6
  Fcn1/1 -> Gain9/1
  Gain8/1 -> Add1/4
  Gain5/1 -> Add1/1
  Fcn3/1 -> Gain6/1
  Fcn4/1 -> Gain7/1
  Gain7/1 -> Add1/3
  Gain11/1 -> Add2/2
  Fcn12/1 -> Gain10/1
  Fcn15/1 -> Gain13/1
  Gain14/1 -> Add2/5
  Fcn13/1 -> Gain11/1
  Gain10/1 -> Add2/1
  Fcn14/1 -> Gain12/1
  Constant2/1 -> Add2/6
  Gain13/1 -> Add2/4
  Fcn11/1 -> Gain14/1
  Gain12/1 -> Add2/3
  Add2/1 -> q3d/1
  Fcn21/1 -> Gain19/1
  Gain19/1 -> Add5/3
  Gain20/1 -> Add5/4
  Fcn18/1 -> Gain21/1
  Gain21/1 -> Add5/5
  Gain18/1 -> Add5/2
  Gain26/1 -> Add4/2
  Fcn23/1 -> Gain25/1
  Fcn26/1 -> Gain28/1
  Constant5/1 -> Add5/6
  Fcn20/1 -> Gain18/1
  Add4/1 -> dq2d/1
  Add3/1 -> dq1d/1
  Add5/1 -> dq3d/1
  Fcn22/1 -> Gain20/1
  Fcn27/1 -> Gain15/1
  Fcn30/1 -> Gain23/1
  Gain17/1 -> Add5/1
  Gain24/1 -> Add3/5
  Constant3/1 -> Add3/6
  Gain16/1 -> Add3/2
  Gain22/1 -> Add3/3
  Fcn19/1 -> Gain17/1
  Gain15/1 -> Add3/1
  Gain23/1 -> Add3/4
  Fcn29/1 -> Gain22/1
  Gain29/1 -> Add4/5
  Fcn17/1 -> Gain24/1
  Fcn24/1 -> Gain26/1
  Gain25/1 -> Add4/1
  Fcn25/1 -> Gain27/1
  Fcn28/1 -> Gain16/1
  Constant4/1 -> Add4/6
  Gain28/1 -> Add4/4
  Fcn16/1 -> Gain29/1
  Gain27/1 -> Add4/3
  Merge/1 -> Fcn33/1, Fcn37/1, Fcn36/1, Fcn35/1, Fcn34/1, Fcn31/1, Fcn41/1, Fcn40/1, Fcn39/1, Fcn38/1, Fcn32/1, Fcn45/1, Fcn44/1, Fcn43/1, Fcn42/1, Fcn18/1, Fcn22/1, Fcn21/1, Fcn20/1, Fcn19/1, Fcn16/1, Fcn26/1, Fcn25/1, Fcn24/1, Fcn23/1, Fcn17/1, Fcn30/1, Fcn29/1, Fcn28/1, Fcn27/1, Fcn11/1, Fcn15/1, Fcn14/1, Fcn13/1, Fcn12/1, Fcn1/1, Fcn5/1, Fcn4/1, Fcn3/1, Fcn2/1, Fcn10/1, Fcn9/1, Fcn8/1, Fcn7/1, Fcn6/1
  Gain32/1 -> Add8/1
  Gain39/1 -> Add6/5
  Constant6/1 -> Add6/6
  Fcn45/1 -> Gain38/1
  Add7/1 -> ddq2d/1
  Fcn42/1 -> Gain30/1
  Add8/1 -> ddq3d/1
  Fcn35/1 -> Gain33/1
  Gain41/1 -> Add7/2
  Fcn37/1 -> Gain35/1
  Gain36/1 -> Add8/5
  Gain35/1 -> Add8/4
  Fcn36/1 -> Gain34/1
  Gain34/1 -> Add8/3
  Fcn33/1 -> Gain36/1
  Gain42/1 -> Add7/3
  Fcn39/1 -> Gain41/1
  Gain33/1 -> Add8/2
  Gain43/1 -> Add7/4
  Add6/1 -> ddq1d/1
  Gain40/1 -> Add7/1
  Constant8/1 -> Add8/6
  Constant7/1 -> Add7/6
  Fcn41/1 -> Gain43/1
  Fcn43/1 -> Gain31/1
  Fcn38/1 -> Gain40/1
  Fcn40/1 -> Gain42/1
  Fcn31/1 -> Gain44/1
  Gain38/1 -> Add6/4
  Fcn44/1 -> Gain37/1
  Fcn34/1 -> Gain32/1
  Gain37/1 -> Add6/3
  Gain30/1 -> Add6/1
  Gain31/1 -> Add6/2
  Gain44/1 -> Add7/5
  Fcn32/1 -> Gain39/1
  Constant9/1 -> If Action Subsystem1/1(In1), If/2
  If/1 -> If Action Subsystem2/Action
  If/2 -> If Action Subsystem1/Action
  If Action Subsystem1/1(Out1) -> Merge/2
  If Action Subsystem2/1(Out1) -> Merge/1
  theta_init/1 -> Terminator1/1
  thetad/1 -> Terminator/1

== system step5_forward_dyn_kine/Trajectory Planning Module1/If Action Subsystem1 ==
  In1 : Inport
  Action Port : ActionPort  ActionPortLabel=else
  Out1 : Outport
  wires:
  In1/1 -> Out1/1

== system step5_forward_dyn_kine/Trajectory Planning Module1/If Action Subsystem2 ==
  In1 : Inport
  Action Port : ActionPort  ActionPortLabel=if(u1 < T_action)
  Out1 : Outport
  wires:
  In1/1 -> Out1/1

== matlab function Disired Forces Computing Module2/MATLAB Function ==
  data: Taud input double; F_cartesian_d output double; qd input double; Rparams input double; F_d output double; thetaF_d output double; Mz_d output double
function [F_cartesian_d, F_d, thetaF_d, Mz_d] = DesiredForcesComputing(Taud,qd,Rparams)

% Rparams4J;
gama1 = Rparams(1);
gama2 = Rparams(2);
gama3 = Rparams(3);
L = Rparams(4);

Rparams4J = [gama1 gama2 gama3];

J = PRBDM_3R_Jacobi(qd,Rparams4J);
J_T = transpose(J);


% F_cartesian = inv(J_T) * Taud;
F_cartesian_d = J_T \ Taud;

FxL = F_cartesian_d(1);
FyL = F_cartesian_d(2);
Mz = F_cartesian_d(3);

thetaF_d = atan2(FyL,FxL);
F_d = FxL/L/cos(thetaF_d);
Mz_d = Mz;

== matlab function Subsystem/MATLAB Function ==
  data: F input double; thetaF input double; Tau1 output double; Mz input double; Rparams input double; q input double; Tau2 output double; Tau3 output double
function [Tau1,Tau2, Tau3] = fcn(F, thetaF, Mz, Rparams, q)

m = Rparams(1);
L = Rparams(2);
gama0 = Rparams(3);
gama1 = Rparams(4);
gama2 = Rparams(5);
gama3 = Rparams(6);


FxL = F*L*cos(thetaF);
FyL = F*L*sin(thetaF);
F_cartesian = [FxL; FyL; Mz];

Rparams4J = zeros(4);
Rparams4J(1) = gama1;
Rparams4J(2) = gama2;
Rparams4J(3) = gama3;
Rparams4J(4) = L;
J = PRBDM_3R_Jacobi(q,Rparams4J);

J_T = transpose(J);

Tau = J_T*F_cartesian;
Tau1 = Tau(1);
Tau2 = Tau(2);
Tau3 = Tau(3);

== matlab function Disired Forces Computing Module1/MATLAB Function ==
  data: Taud input double; F_cartesian_d output double; qd input double; Rparams input double; F_d output double; thetaF_d output double; Mz_d output double
function [F_cartesian_d, F_d, thetaF_d, Mz_d] = DesiredForcesComputing(Taud,qd,Rparams)

% Rparams4J;
gama1 = Rparams(1);
gama2 = Rparams(2);
gama3 = Rparams(3);
L = Rparams(4);

Rparams4J = [gama1 gama2 gama3];

J = PRBDM_3R_Jacobi(qd,Rparams4J);
J_T = transpose(J);


% F_cartesian = inv(J_T) * Taud;
F_cartesian_d = J_T \ Taud;

FxL = F_cartesian_d(1);
FyL = F_cartesian_d(2);
Mz = F_cartesian_d(3);

thetaF_d = atan2(FyL,FxL);
F_d = FxL/L/cos(thetaF_d);
Mz_d = Mz;

== matlab function Inverse Dynamics Module1/TorqueComputing ==
  data: qd input double; Taud output double; dqd input double; ddqd input double; Rparams input double
function Taud = DisiredTorqueComputing(qd, dqd, ddqd, Rparams)

q1d = qd(1);
q2d = qd(2);
q3d = qd(3);

dq1d = dqd(1);
dq2d = dqd(2);
dq3d = dqd(3);

ddq1d = ddqd(1);
ddq2d = ddqd(2);
ddq3d = ddqd(3);

m = Rparams(1);
L = Rparams(2);
gama0 = Rparams(3);
gama1 = Rparams(4);
gama2 = Rparams(5);
gama3 = Rparams(6);
k1 = Rparams(7);
k2 = Rparams(8);
k3 = Rparams(9);
I = Rparams(10);


robot_params = zeros(7);
robot_params(1) = m;
robot_params(2) = L;
robot_params(3) = gama0;
robot_params(4) = gama1;
robot_params(5) = gama2;
robot_params(6) = gama3;
robot_params(7) = I;

[A,B,C,D] = PRBDM_3R_Dynamic_Matrices_Lagrange(qd,robot_params);

dqid = [dq1d;dq1d;dq2d];
dqjd = [dq2d;dq3d;dq3d]; 
dqid_dqjd = dqid.*dqjd;
Taud = A*ddqd + B*(dqd.^2) + C*dqid_dqjd + D*qd;
